simulink model "graphical_function2_2018a"  (R2018a)
settings: Solver=VariableStepAuto  StartTime=0.0  StopTime=10.0  RelTol=1e-3
settings Model: Creator=86188  LastModifiedBy=86188

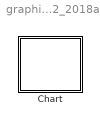
== system graphical_function2_2018a ==
  Chart : Stateflow chart  TreatAsAtomicUnit=on

== stateflow chart graphical_function2_2018a/Chart ==
  state i=set_message(sn) [function]
    (junction 10) -> (junction 4) : {buffer_data(WriterId,i)=WHC(sn);i = i + 1;f("set_mesg")}
    (junction 4) -> (junction 3)
    (junction 3) -> (junction 10) [order 1] : [i<=2]
    (default) -> (junction 3) : {i=1}
    (junction 3) -> (junction 9) [order 2]
  state A
    en: f("en_A");
    data=set_message(1)
  state B
    en: f("en_B")
  (default) -> A
  A -> B
  data: sn function_input; i function_output; s function_input; WHC local size=[1 5] =[100 200 300 400 500]; buffer_data local size=[2 2] =[0 0;0 0]; WriterId local =1; data local =0
  function f(s):
    | function f(s)
    |   fprintf(s+"\n");
